simulink library "forward_dynamics_v1"  (R2020b)
settings: Solver=VariableStepAuto  StartTime=0.0  StopTime=10.0  RelTol=1e-3
undefined symbols (not defined in the file): Config, DiscIntNeverNeededParam
libraries: WBToolboxLibrary x21
settings Model: Creator=gnava  LastModifiedBy=gnava

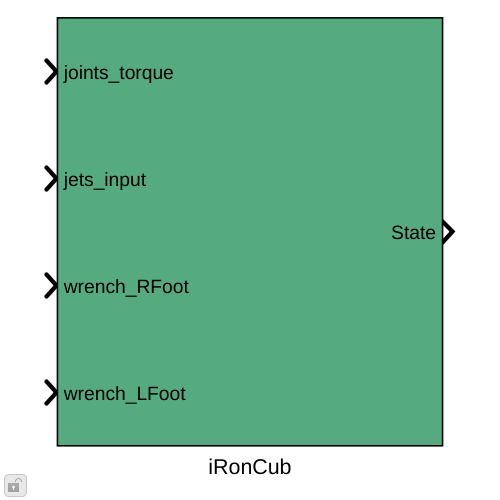
[thumbnail: Simulink's stored preview of the top-level diagram]
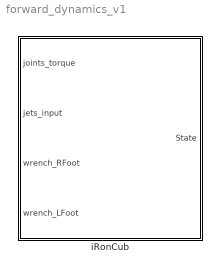
== system forward_dynamics_v1 ==
  iRonCub : Subsystem  mask{Config=Config}
      mask prompts: Config "Configuration structure"
      mask DialogControl DescTextVar Prompt: Block that simulates iRonCub

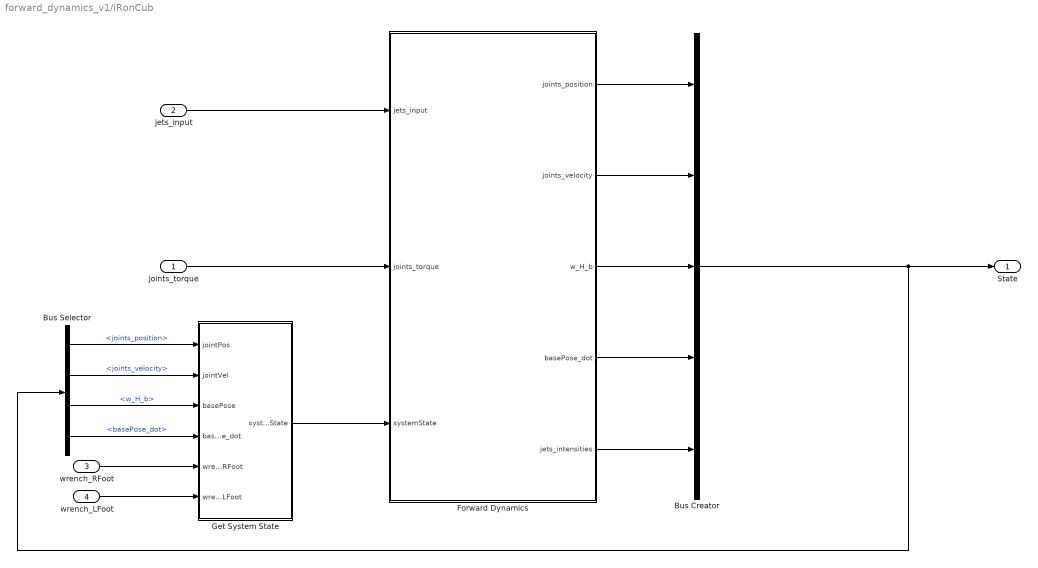
== system forward_dynamics_v1/iRonCub ==
  joints_torque : Inport
  jets_input : Inport  Port=2
  wrench_RFoot : Inport  Port=3
  wrench_LFoot : Inport  Port=4
  Bus Creator : BusCreator  Inputs=5
  Bus Selector : BusSelector  OutputSignals=joints_position,joints_velocity,w_H_b,basePose_dot
  Forward Dynamics : Subsystem
  Get System State : Subsystem
  State : Outport  VectorParamsAs1DForOutWhenUnconnected=off
  wires:
  jets_input/1 -> Forward Dynamics/1(jets_input)
  Get System State/1(systemState) -> Forward Dynamics/3(systemState)
  joints_torque/1 -> Forward Dynamics/2(joints_torque)
  Forward Dynamics/1(joints_position) -> Bus Creator/1
  Forward Dynamics/3(w_H_b) -> Bus Creator/3
  Forward Dynamics/4(basePose_dot) -> Bus Creator/4
  Bus Creator/1 -> State/1, Bus Selector/1
  Bus Selector/1 -> Get System State/1(jointPos)  "<joints_position>"
  Bus Selector/2 -> Get System State/2(jointVel)  "<joints_velocity>"
  Bus Selector/3 -> Get System State/3(basePose)  "<w_H_b>"
  Bus Selector/4 -> Get System State/4(basePose_dot)  "<basePose_dot>"
  wrench_RFoot/1 -> Get System State/5(wrench_RFoot)
  wrench_LFoot/1 -> Get System State/6(wrench_LFoot)
  Forward Dynamics/5(jets_intensities) -> Bus Creator/5
  Forward Dynamics/2(joints_velocity) -> Bus Creator/2

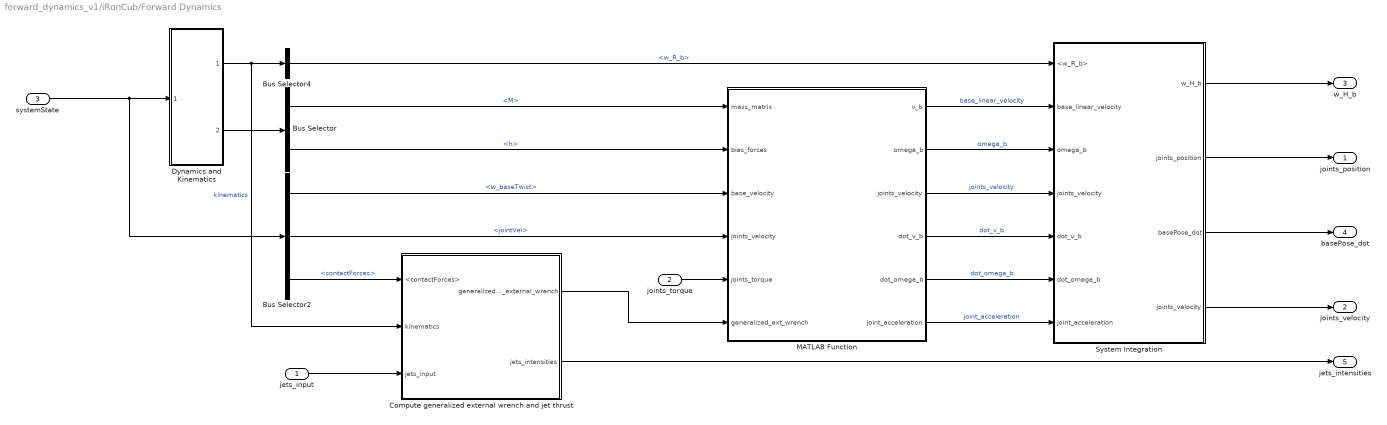
== system forward_dynamics_v1/iRonCub/Forward Dynamics ==
  jets_input : Inport
  joints_torque : Inport  Port=2
  systemState : Inport  Port=3
  Bus Selector : BusSelector  OutputSignals=M,h
  Bus Selector2 : BusSelector  OutputSignals=w_baseTwist,jointVel,contactForces
  Bus Selector4 : BusSelector  OutputSignals=w_R_b
  Compute generalized external wrench and jet thrust : Subsystem
  Dynamics and Kinematics : Subsystem
  MATLAB Function : MATLAB Function  TreatAsAtomicUnit=on
  System Integration : Subsystem
  joints_position : Outport  VectorParamsAs1DForOutWhenUnconnected=off
  joints_velocity : Outport  Port=2  VectorParamsAs1DForOutWhenUnconnected=off
  w_H_b : Outport  Port=3  VectorParamsAs1DForOutWhenUnconnected=off
  basePose_dot : Outport  Port=4  VectorParamsAs1DForOutWhenUnconnected=off
  jets_intensities : Outport  Port=5  VectorParamsAs1DForOutWhenUnconnected=off
  wires:
  Dynamics and Kinematics/1(kinematics) -> Compute generalized external wrench and jet thrust/2(kinematics), Bus Selector4/1  "kinematics"
  Bus Selector/2 -> MATLAB Function/2(bias_forces)  "<h>"
  Bus Selector/1 -> MATLAB Function/1(mass_matrix)  "<M>"
  Bus Selector2/1 -> MATLAB Function/3(base_velocity)  "<w_baseTwist>"
  Dynamics and Kinematics/2(dynamics) -> Bus Selector/1
  Bus Selector2/2 -> MATLAB Function/4("joints_velocity ")  "<jointVel>"
  systemState/1 -> Bus Selector2/1, Dynamics and Kinematics/1(systemState)
  MATLAB Function/1(v_b) -> System Integration/2(base_linear_velocity)  "base_linear_velocity"
  MATLAB Function/2(omega_b) -> System Integration/3(omega_b)  "omega_b"
  MATLAB Function/3(joints_velocity) -> System Integration/4(joints_velocity)  "joints_velocity"
  MATLAB Function/4(dot_v_b) -> System Integration/5(dot_v_b)  "dot_v_b"
  MATLAB Function/5(dot_omega_b) -> System Integration/6(dot_omega_b)  "dot_omega_b"
  MATLAB Function/6(joint_acceleration) -> System Integration/7(joint_acceleration)  "joint_acceleration"
  System Integration/1(w_H_b) -> w_H_b/1
  System Integration/2(joints_position) -> joints_position/1
  System Integration/3(basePose_dot) -> basePose_dot/1
  System Integration/4("joints_velocity ") -> joints_velocity/1
  Bus Selector4/1 -> System Integration/1(<w_R_b>)  "<w_R_b>"
  joints_torque/1 -> MATLAB Function/5(joints_torque)
  Bus Selector2/3 -> Compute generalized external wrench and jet thrust/1(<contactForces>)  "<contactForces>"
  jets_input/1 -> Compute generalized external wrench and jet thrust/3(jets_input)
  Compute generalized external wrench and jet thrust/1(generalized_external_wrench) -> MATLAB Function/6(generalized_ext_wrench)
  Compute generalized external wrench and jet thrust/2(jets_intensities) -> jets_intensities/1

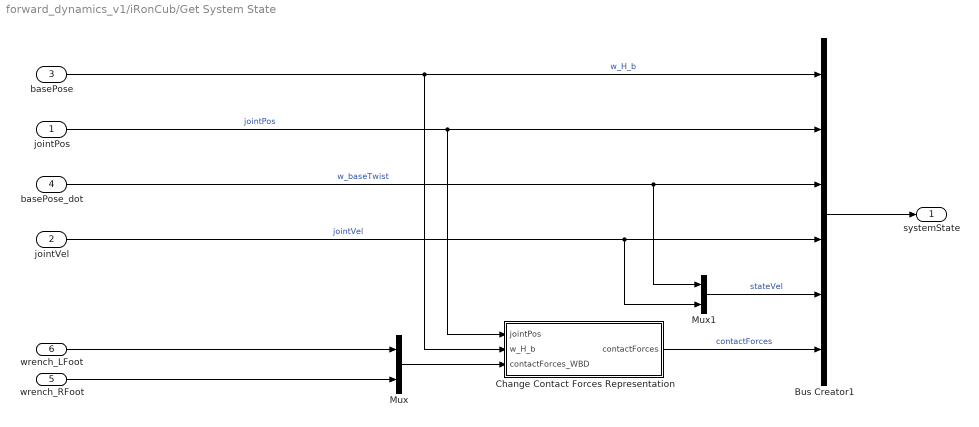
== system forward_dynamics_v1/iRonCub/Get System State ==
  jointPos : Inport
  jointVel : Inport  Port=2
  basePose : Inport  Port=3
  basePose_dot : Inport  Port=4
  wrench_RFoot : Inport  Port=5
  wrench_LFoot : Inport  Port=6
  Bus Creator1 : BusCreator  Inputs=6
  Change Contact Forces Representation : Subsystem
  Mux : Mux  Inputs=2
  Mux1 : Mux  Inputs=2
  systemState : Outport  VectorParamsAs1DForOutWhenUnconnected=off
  wires:
  wrench_LFoot/1 -> Mux/1
  wrench_RFoot/1 -> Mux/2
  Mux/1 -> Change Contact Forces Representation/3(contactForces_WBD)
  Change Contact Forces Representation/1(contactForces) -> Bus Creator1/6  "contactForces"
  jointVel/1 -> Bus Creator1/4, Mux1/2  "jointVel"
  Bus Creator1/1 -> systemState/1
  Mux1/1 -> Bus Creator1/5  "stateVel"
  basePose_dot/1 -> Bus Creator1/3, Mux1/1  "w_baseTwist"
  jointPos/1 -> Bus Creator1/2, Change Contact Forces Representation/1(jointPos)  "jointPos"
  basePose/1 -> Change Contact Forces Representation/2(w_H_b), Bus Creator1/1  "w_H_b"

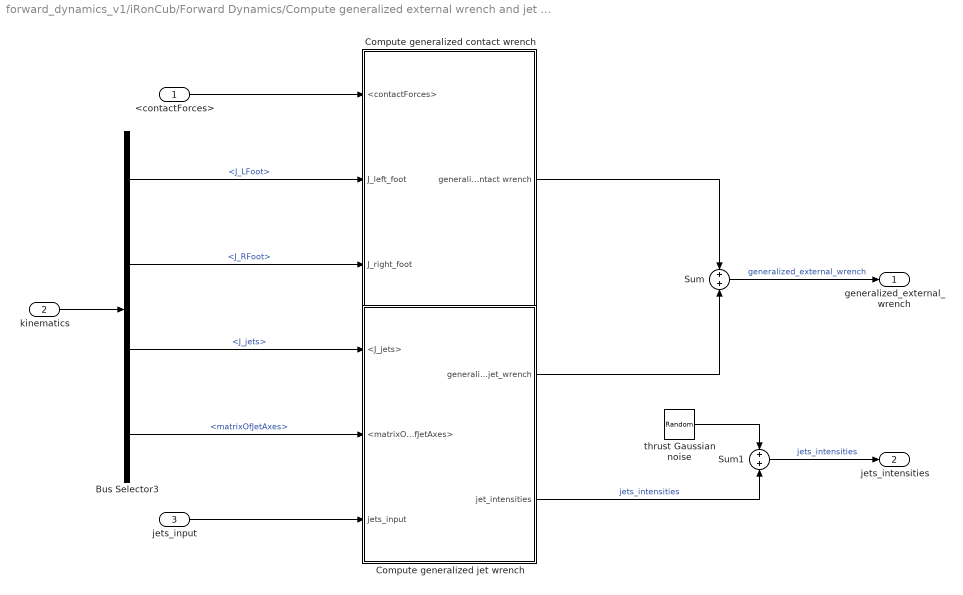
== system forward_dynamics_v1/iRonCub/Forward Dynamics/Compute generalized external wrench and jet thrust ==
  <contactForces> : Inport
  kinematics : Inport  Port=2
  jets_input : Inport  Port=3
  Bus Selector3 : BusSelector  OutputSignals=J_LFoot,J_RFoot,J_jets,matrixOfJetAxes
  "Compute generalized contact wrench " : Subsystem
  Compute generalized jet wrench : Subsystem
  Sum : Sum
  Sum1 : Sum
  "thrust Gaussian noise " : RandomNumber  Variance=Config.thrust_noise
  generalized_external_wrench : Outport  VectorParamsAs1DForOutWhenUnconnected=off
  jets_intensities : Outport  Port=2  VectorParamsAs1DForOutWhenUnconnected=off
  wires:
  Sum1/1 -> jets_intensities/1  "jets_intensities"
  "Compute generalized contact wrench "/1("generalized contact wrench ") -> Sum/1
  Bus Selector3/4 -> Compute generalized jet wrench/2(<matrixOfJetAxes>)  "<matrixOfJetAxes>"
  jets_input/1 -> Compute generalized jet wrench/3(jets_input)
  Bus Selector3/3 -> Compute generalized jet wrench/1(<J_jets>)  "<J_jets>"
  kinematics/1 -> Bus Selector3/1
  Compute generalized jet wrench/1(generalized_jet_wrench) -> Sum/2
  <contactForces>/1 -> "Compute generalized contact wrench "/1(<contactForces>)
  Sum/1 -> generalized_external_wrench/1  "generalized_external_wrench"
  Bus Selector3/1 -> "Compute generalized contact wrench "/2(J_left_foot)  "<J_LFoot>"
  Bus Selector3/2 -> "Compute generalized contact wrench "/3(J_right_foot)  "<J_RFoot>"
  "thrust Gaussian noise "/1 -> Sum1/1
  Compute generalized jet wrench/2(jet_intensities) -> Sum1/2  "jets_intensities"

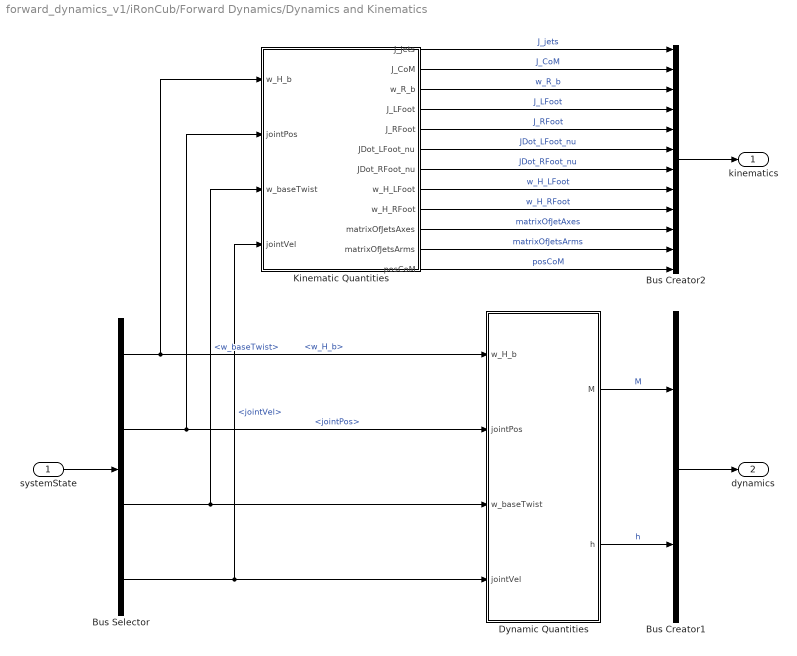
== system forward_dynamics_v1/iRonCub/Forward Dynamics/Dynamics and Kinematics ==
  systemState : Inport
  Bus Creator1 : BusCreator  Inputs=2
  Bus Creator2 : BusCreator  Inputs=12
  Bus Selector : BusSelector  OutputSignals=w_H_b,jointPos,w_baseTwist,jointVel
  Dynamic Quantities : Subsystem
  Kinematic Quantities : Subsystem
  kinematics : Outport  VectorParamsAs1DForOutWhenUnconnected=off
  dynamics : Outport  Port=2  VectorParamsAs1DForOutWhenUnconnected=off
  wires:
  systemState/1 -> Bus Selector/1
  Bus Selector/1 -> Dynamic Quantities/1(w_H_b), Kinematic Quantities/1(w_H_b)  "<w_H_b>"
  Bus Selector/2 -> Kinematic Quantities/2(jointPos), Dynamic Quantities/2(jointPos)  "<jointPos>"
  Bus Selector/3 -> Kinematic Quantities/3(w_baseTwist), Dynamic Quantities/3(w_baseTwist)  "<w_baseTwist>"
  Bus Selector/4 -> Kinematic Quantities/4(jointVel), Dynamic Quantities/4(jointVel)  "<jointVel>"
  Dynamic Quantities/2("h ") -> Bus Creator1/2  "h"
  Dynamic Quantities/1(M) -> Bus Creator1/1  "M"
  Bus Creator1/1 -> dynamics/1
  Bus Creator2/1 -> kinematics/1
  Kinematic Quantities/1(J_jets) -> Bus Creator2/1  "J_jets"
  Kinematic Quantities/2(J_CoM) -> Bus Creator2/2  "J_CoM"
  Kinematic Quantities/3(w_R_b) -> Bus Creator2/3  "w_R_b"
  Kinematic Quantities/4(J_LFoot) -> Bus Creator2/4  "J_LFoot"
  Kinematic Quantities/5(J_RFoot) -> Bus Creator2/5  "J_RFoot"
  Kinematic Quantities/6(JDot_LFoot_nu) -> Bus Creator2/6  "JDot_LFoot_nu"
  Kinematic Quantities/7(JDot_RFoot_nu) -> Bus Creator2/7  "JDot_RFoot_nu"
  Kinematic Quantities/8(w_H_LFoot) -> Bus Creator2/8  "w_H_LFoot"
  Kinematic Quantities/9(w_H_RFoot) -> Bus Creator2/9  "w_H_RFoot"
  Kinematic Quantities/10(matrixOfJetsAxes) -> Bus Creator2/10  "matrixOfJetAxes"
  Kinematic Quantities/11(matrixOfJetsArms) -> Bus Creator2/11  "matrixOfJetsArms"
  Kinematic Quantities/12(posCoM) -> Bus Creator2/12  "posCoM"

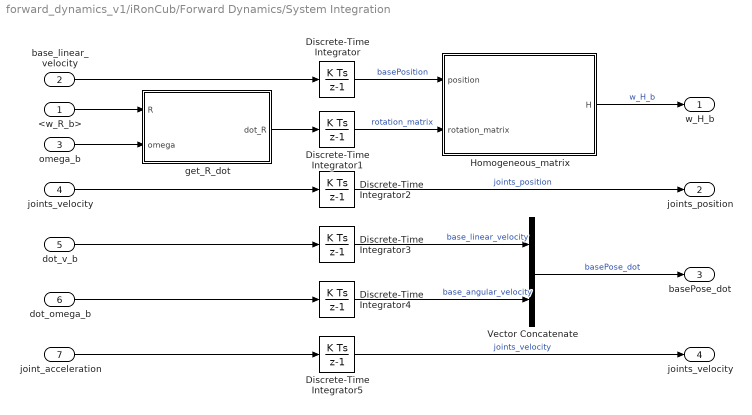
== system forward_dynamics_v1/iRonCub/Forward Dynamics/System Integration ==
  <w_R_b> : Inport
  base_linear_velocity : Inport  Port=2
  omega_b : Inport  Port=3
  joints_velocity : Inport  Port=4
  dot_v_b : Inport  Port=5
  dot_omega_b : Inport  Port=6
  joint_acceleration : Inport  Port=7
  Discrete-Time Integrator : DiscreteIntegrator  InitialCondition=Config.initialConditions.base_position  SampleTime=-1  ICPrevOutput=DiscIntNeverNeededParam  ICPrevScaledInput=DiscIntNeverNeededParam
  Discrete-Time Integrator1 : DiscreteIntegrator  InitialCondition=Config.initialConditions.orientation  SampleTime=-1  ICPrevOutput=DiscIntNeverNeededParam  ICPrevScaledInput=DiscIntNeverNeededParam
  Discrete-Time Integrator2 : DiscreteIntegrator  InitialCondition=Config.initialConditions.joints  SampleTime=-1  ICPrevOutput=DiscIntNeverNeededParam  ICPrevScaledInput=DiscIntNeverNeededParam
  Discrete-Time Integrator3 : DiscreteIntegrator  InitialCondition=Config.initialConditions.base_linear_velocity  SampleTime=-1  ICPrevOutput=DiscIntNeverNeededParam  ICPrevScaledInput=DiscIntNeverNeededParam
  Discrete-Time Integrator4 : DiscreteIntegrator  InitialCondition=Config.initialConditions.base_angular_velocity  SampleTime=-1  ICPrevOutput=DiscIntNeverNeededParam  ICPrevScaledInput=DiscIntNeverNeededParam
  Discrete-Time Integrator5 : DiscreteIntegrator  InitialCondition=Config.initialConditions.joints_velocity  SampleTime=-1  ICPrevOutput=DiscIntNeverNeededParam  ICPrevScaledInput=DiscIntNeverNeededParam
  "Homogeneous_matrix " : MATLAB Function  TreatAsAtomicUnit=on
  Vector Concatenate : Concatenate
  "get_R_dot " : MATLAB Function  TreatAsAtomicUnit=on
  w_H_b : Outport  VectorParamsAs1DForOutWhenUnconnected=off
  joints_position : Outport  Port=2  VectorParamsAs1DForOutWhenUnconnected=off
  basePose_dot : Outport  Port=3  VectorParamsAs1DForOutWhenUnconnected=off
  "joints_velocity " : Outport  Port=4  VectorParamsAs1DForOutWhenUnconnected=off
  wires:
  Discrete-Time Integrator3/1 -> Vector Concatenate/1  "base_linear_velocity"
  omega_b/1 -> "get_R_dot "/2(omega)
  Discrete-Time Integrator5/1 -> "joints_velocity "/1  "joints_velocity"
  dot_v_b/1 -> Discrete-Time Integrator3/1
  Discrete-Time Integrator2/1 -> joints_position/1  "joints_position"
  <w_R_b>/1 -> "get_R_dot "/1(R)
  Discrete-Time Integrator4/1 -> Vector Concatenate/2  "base_angular_velocity"
  "Homogeneous_matrix "/1(H) -> w_H_b/1  "w_H_b"
  Vector Concatenate/1 -> basePose_dot/1  "basePose_dot"
  joints_velocity/1 -> Discrete-Time Integrator2/1
  Discrete-Time Integrator/1 -> "Homogeneous_matrix "/1(position)  "basePosition"
  base_linear_velocity/1 -> Discrete-Time Integrator/1
  "get_R_dot "/1(dot_R) -> Discrete-Time Integrator1/1
  dot_omega_b/1 -> Discrete-Time Integrator4/1
  joint_acceleration/1 -> Discrete-Time Integrator5/1
  Discrete-Time Integrator1/1 -> "Homogeneous_matrix "/2(rotation_matrix)  "rotation_matrix"

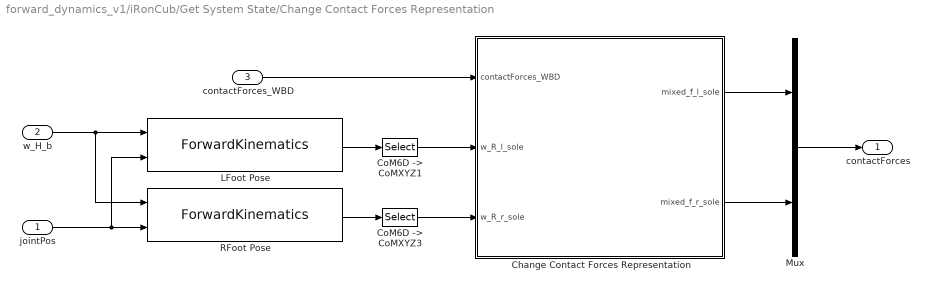
== system forward_dynamics_v1/iRonCub/Get System State/Change Contact Forces Representation ==
  jointPos : Inport
  w_H_b : Inport  Port=2
  contactForces_WBD : Inport  Port=3
  Change Contact Forces Representation : MATLAB Function  TreatAsAtomicUnit=on
  "CoM6D -> CoMXYZ1" : Selector  NumberOfDimensions=2  InputPortWidth=7  IndexOptions=Index vector (dialog),Index vector (dialog)  Indices=[1 2 3],[1 2 3]  OutputSizes=1,1
  "CoM6D -> CoMXYZ3" : Selector  NumberOfDimensions=2  InputPortWidth=7  IndexOptions=Index vector (dialog),Index vector (dialog)  Indices=[1 2 3],[1 2 3]  OutputSizes=1,1
  LFoot Pose : WBToolboxLibrary/Model/Kinematics/ForwardKinematics  frameName=Frames.LFOOT_FRAME
      settings: SourceProductName=WholeBodyToolbox
  Mux : Mux  Inputs=2
  RFoot Pose : WBToolboxLibrary/Model/Kinematics/ForwardKinematics  frameName=Frames.RFOOT_FRAME
      settings: SourceProductName=WholeBodyToolbox
  contactForces : Outport  VectorParamsAs1DForOutWhenUnconnected=off
  wires:
  contactForces_WBD/1 -> Change Contact Forces Representation/1(contactForces_WBD)
  RFoot Pose/1 -> "CoM6D -> CoMXYZ3"/1
  "CoM6D -> CoMXYZ3"/1 -> Change Contact Forces Representation/3(w_R_r_sole)
  LFoot Pose/1 -> "CoM6D -> CoMXYZ1"/1
  "CoM6D -> CoMXYZ1"/1 -> Change Contact Forces Representation/2(w_R_l_sole)
  w_H_b/1 -> LFoot Pose/1, RFoot Pose/1
  jointPos/1 -> LFoot Pose/2, RFoot Pose/2
  Change Contact Forces Representation/1(mixed_f_l_sole) -> Mux/1
  Change Contact Forces Representation/2(mixed_f_r_sole) -> Mux/2
  Mux/1 -> contactForces/1

== system forward_dynamics_v1/iRonCub/Forward Dynamics/Compute generalized external wrench and jet thrust/Compute generalized contact wrench  ==
  <contactForces> : Inport
  J_left_foot : Inport  Port=2
  J_right_foot : Inport  Port=3
  Matrix Concatenate : Concatenate  Mode=Multidimensional array
  MatrixMultiply : Product  Multiplication=Matrix(*)
  Transpose : Math  Operator=transpose  SignedPower=on  SaturateOnIntegerOverflow=on
  "generalized contact wrench " : Outport  VectorParamsAs1DForOutWhenUnconnected=off
  wires:
  J_left_foot/1 -> Matrix Concatenate/1
  J_right_foot/1 -> Matrix Concatenate/2
  Matrix Concatenate/1 -> Transpose/1
  <contactForces>/1 -> MatrixMultiply/2
  Transpose/1 -> MatrixMultiply/1
  MatrixMultiply/1 -> "generalized contact wrench "/1

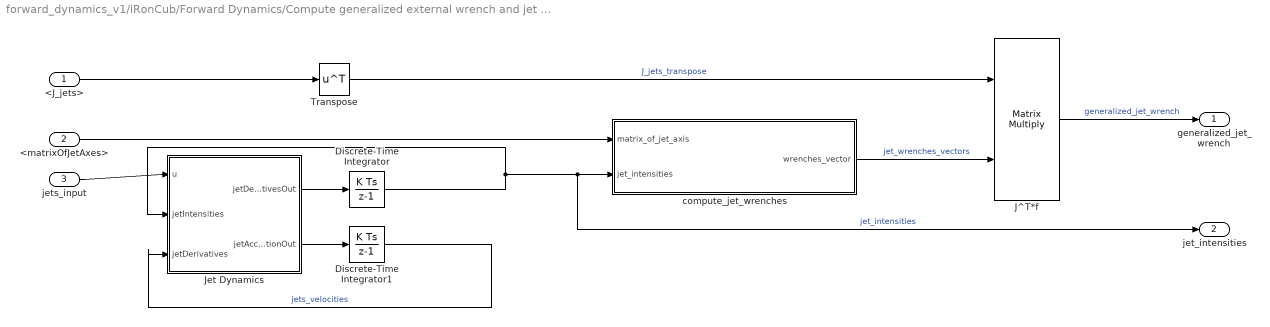
== system forward_dynamics_v1/iRonCub/Forward Dynamics/Compute generalized external wrench and jet thrust/Compute generalized jet wrench ==
  <J_jets> : Inport
  <matrixOfJetAxes> : Inport  Port=2
  jets_input : Inport  Port=3
  Discrete-Time Integrator : DiscreteIntegrator  InitialCondition=Config.initialConditions.jets_thrust  SampleTime=-1  ICPrevOutput=DiscIntNeverNeededParam  ICPrevScaledInput=DiscIntNeverNeededParam
  Discrete-Time Integrator1 : DiscreteIntegrator  SampleTime=-1  ICPrevOutput=DiscIntNeverNeededParam  ICPrevScaledInput=DiscIntNeverNeededParam
  J^T*f : Product  Multiplication=Matrix(*)
  Jet Dynamics : MATLAB Function  TreatAsAtomicUnit=on
  Transpose : Math  Operator=transpose  SignedPower=on  SaturateOnIntegerOverflow=on
  "compute_jet_wrenches " : MATLAB Function  TreatAsAtomicUnit=on
  generalized_jet_wrench : Outport  VectorParamsAs1DForOutWhenUnconnected=off
  jet_intensities : Outport  Port=2  VectorParamsAs1DForOutWhenUnconnected=off
  wires:
  "compute_jet_wrenches "/1(wrenches_vector) -> J^T*f/2  "jet_wrenches_vectors"
  <matrixOfJetAxes>/1 -> "compute_jet_wrenches "/1(matrix_of_jet_axis)
  Transpose/1 -> J^T*f/1  "J_jets_transpose"
  <J_jets>/1 -> Transpose/1
  jets_input/1 -> Jet Dynamics/1(u)
  Discrete-Time Integrator/1 -> jet_intensities/1, "compute_jet_wrenches "/2(jet_intensities), Jet Dynamics/2(jetIntensities)  "jet_intensities"
  J^T*f/1 -> generalized_jet_wrench/1  "generalized_jet_wrench"
  Jet Dynamics/2(jetAccelerationOut) -> Discrete-Time Integrator1/1
  Discrete-Time Integrator1/1 -> Jet Dynamics/3(jetDerivatives)  "jets_velocities"
  Jet Dynamics/1(jetDerivativesOut) -> Discrete-Time Integrator/1

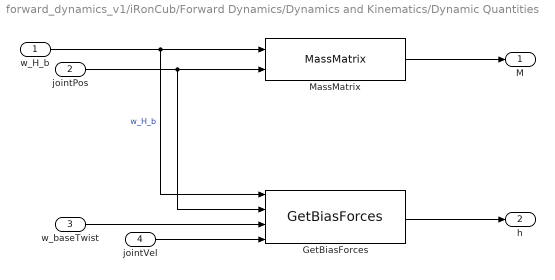
== system forward_dynamics_v1/iRonCub/Forward Dynamics/Dynamics and Kinematics/Dynamic Quantities ==
  w_H_b : Inport
  jointPos : Inport  Port=2
  w_baseTwist : Inport  Port=3
  jointVel : Inport  Port=4
  GetBiasForces : WBToolboxLibrary/Model/Dynamics/GetBiasForces
      settings: SourceProductName=WholeBodyToolbox
  MassMatrix : WBToolboxLibrary/Model/Dynamics/MassMatrix
      settings: SourceProductName=WholeBodyToolbox
  M : Outport  VectorParamsAs1DForOutWhenUnconnected=off
  "h " : Outport  Port=2  VectorParamsAs1DForOutWhenUnconnected=off
  wires:
  w_H_b/1 -> GetBiasForces/1, MassMatrix/1  "w_H_b"
  w_baseTwist/1 -> GetBiasForces/3
  jointVel/1 -> GetBiasForces/4
  MassMatrix/1 -> M/1
  GetBiasForces/1 -> "h "/1
  jointPos/1 -> GetBiasForces/2, MassMatrix/2

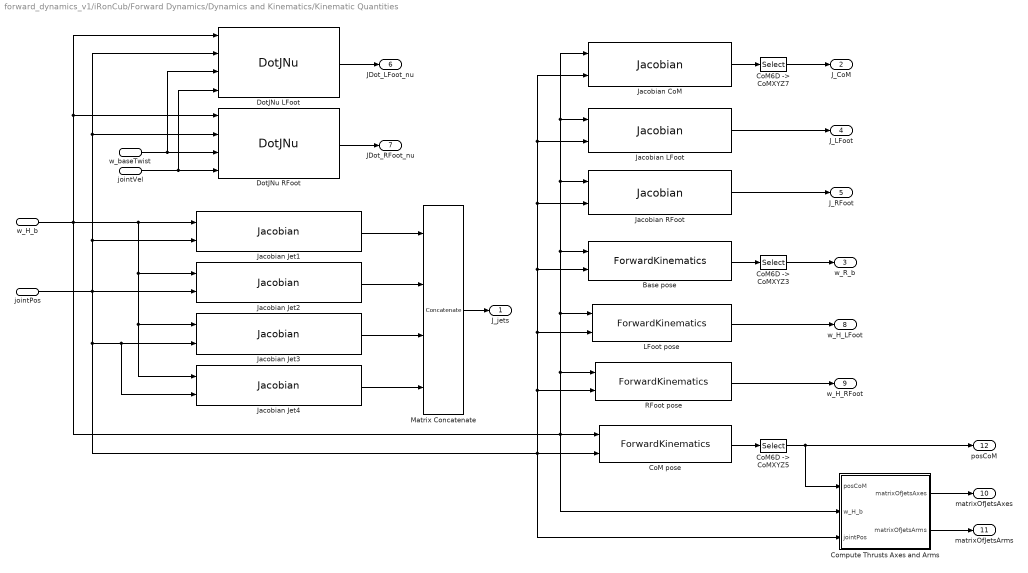
== system forward_dynamics_v1/iRonCub/Forward Dynamics/Dynamics and Kinematics/Kinematic Quantities ==
  w_H_b : Inport
  jointPos : Inport  Port=2
  w_baseTwist : Inport  Port=3
  jointVel : Inport  Port=4
  Base pose : WBToolboxLibrary/Model/Kinematics/ForwardKinematics  frameName=Frames.BASE_LINK
      settings: SourceProductName=WholeBodyToolbox
  CoM pose : WBToolboxLibrary/Model/Kinematics/ForwardKinematics  frameName=Frames.COM_FRAME
      settings: SourceProductName=WholeBodyToolbox
  "CoM6D -> CoMXYZ3" : Selector  NumberOfDimensions=2  InputPortWidth=7  IndexOptions=Index vector (dialog),Index vector (dialog)  Indices=[1 2 3],[1 2 3]  OutputSizes=1,1
  "CoM6D -> CoMXYZ5" : Selector  NumberOfDimensions=2  InputPortWidth=7  IndexOptions=Index vector (dialog),Index vector (dialog)  Indices=[1 2 3],[4]  OutputSizes=1,1
  "CoM6D -> CoMXYZ7" : Selector  NumberOfDimensions=2  InputPortWidth=7  IndexOptions=Index vector (dialog),Index vector (dialog)  Indices=[1 2 3],[1:6+Config.N_DOF]  OutputSizes=1,1
  Compute Thrusts Axes and Arms : Subsystem
  DotJNu LFoot : WBToolboxLibrary/Model/Jacobians/DotJNu  frameName=Frames.LFOOT_FRAME
      settings: SourceProductName=WholeBodyToolbox
  DotJNu RFoot : WBToolboxLibrary/Model/Jacobians/DotJNu  frameName=Frames.RFOOT_FRAME
      settings: SourceProductName=WholeBodyToolbox
  Jacobian CoM : WBToolboxLibrary/Model/Jacobians/Jacobian  frameName=Frames.COM_FRAME
      settings: SourceProductName=WholeBodyToolbox
  Jacobian Jet1 : WBToolboxLibrary/Model/Jacobians/Jacobian  frameName=Frames.JET1_FRAME
      settings: SourceProductName=WholeBodyToolbox
  Jacobian Jet2 : WBToolboxLibrary/Model/Jacobians/Jacobian  frameName=Frames.JET2_FRAME
      settings: SourceProductName=WholeBodyToolbox
  Jacobian Jet3 : WBToolboxLibrary/Model/Jacobians/Jacobian  frameName=Frames.JET3_FRAME
      settings: SourceProductName=WholeBodyToolbox
  Jacobian Jet4 : WBToolboxLibrary/Model/Jacobians/Jacobian  frameName=Frames.JET4_FRAME
      settings: SourceProductName=WholeBodyToolbox
  Jacobian LFoot : WBToolboxLibrary/Model/Jacobians/Jacobian  frameName=Frames.LFOOT_FRAME
      settings: SourceProductName=WholeBodyToolbox
  Jacobian RFoot : WBToolboxLibrary/Model/Jacobians/Jacobian  frameName=Frames.RFOOT_FRAME
      settings: SourceProductName=WholeBodyToolbox
  LFoot pose : WBToolboxLibrary/Model/Kinematics/ForwardKinematics  frameName=Frames.LFOOT_FRAME
      settings: SourceProductName=WholeBodyToolbox
  Matrix Concatenate : Concatenate  NumInputs=4  Mode=Multidimensional array
  RFoot pose : WBToolboxLibrary/Model/Kinematics/ForwardKinematics  frameName=Frames.RFOOT_FRAME
      settings: SourceProductName=WholeBodyToolbox
  J_jets : Outport  VectorParamsAs1DForOutWhenUnconnected=off
  J_CoM : Outport  Port=2  VectorParamsAs1DForOutWhenUnconnected=off
  w_R_b : Outport  Port=3  VectorParamsAs1DForOutWhenUnconnected=off
  J_LFoot : Outport  Port=4  VectorParamsAs1DForOutWhenUnconnected=off
  J_RFoot : Outport  Port=5  VectorParamsAs1DForOutWhenUnconnected=off
  JDot_LFoot_nu : Outport  Port=6  VectorParamsAs1DForOutWhenUnconnected=off
  JDot_RFoot_nu : Outport  Port=7  VectorParamsAs1DForOutWhenUnconnected=off
  w_H_LFoot : Outport  Port=8  VectorParamsAs1DForOutWhenUnconnected=off
  w_H_RFoot : Outport  Port=9  VectorParamsAs1DForOutWhenUnconnected=off
  matrixOfJetsAxes : Outport  Port=10  VectorParamsAs1DForOutWhenUnconnected=off
  matrixOfJetsArms : Outport  Port=11  VectorParamsAs1DForOutWhenUnconnected=off
  posCoM : Outport  Port=12  VectorParamsAs1DForOutWhenUnconnected=off
  wires:
  Matrix Concatenate/1 -> J_jets/1
  CoM pose/1 -> "CoM6D -> CoMXYZ5"/1
  "CoM6D -> CoMXYZ5"/1 -> posCoM/1, Compute Thrusts Axes and Arms/1(posCoM)
  w_H_b/1 -> LFoot pose/1, Base pose/1, Jacobian LFoot/1, Jacobian CoM/1, Jacobian RFoot/1, RFoot pose/1, CoM pose/1, Compute Thrusts Axes and Arms/2(w_H_b), DotJNu LFoot/1, DotJNu RFoot/1, Jacobian Jet4/1, Jacobian Jet3/1, Jacobian Jet2/1, Jacobian Jet1/1
  "CoM6D -> CoMXYZ3"/1 -> w_R_b/1
  jointPos/1 -> Jacobian Jet4/2, Jacobian Jet3/2, Compute Thrusts Axes and Arms/3(jointPos), LFoot pose/2, Jacobian RFoot/2, Jacobian LFoot/2, Jacobian CoM/2, Base pose/2, RFoot pose/2, CoM pose/2, Jacobian Jet2/2, DotJNu LFoot/2, DotJNu RFoot/2, Jacobian Jet1/2
  Jacobian CoM/1 -> "CoM6D -> CoMXYZ7"/1
  Jacobian RFoot/1 -> J_RFoot/1
  Jacobian LFoot/1 -> J_LFoot/1
  DotJNu RFoot/1 -> JDot_RFoot_nu/1
  DotJNu LFoot/1 -> JDot_LFoot_nu/1
  jointVel/1 -> DotJNu RFoot/4, DotJNu LFoot/4
  w_baseTwist/1 -> DotJNu LFoot/3, DotJNu RFoot/3
  RFoot pose/1 -> w_H_RFoot/1
  LFoot pose/1 -> w_H_LFoot/1
  Base pose/1 -> "CoM6D -> CoMXYZ3"/1
  Compute Thrusts Axes and Arms/2(matrixOfJetsArms) -> matrixOfJetsArms/1
  Compute Thrusts Axes and Arms/1(matrixOfJetsAxes) -> matrixOfJetsAxes/1
  Jacobian Jet1/1 -> Matrix Concatenate/1
  Jacobian Jet2/1 -> Matrix Concatenate/2
  Jacobian Jet3/1 -> Matrix Concatenate/3
  Jacobian Jet4/1 -> Matrix Concatenate/4
  "CoM6D -> CoMXYZ7"/1 -> J_CoM/1

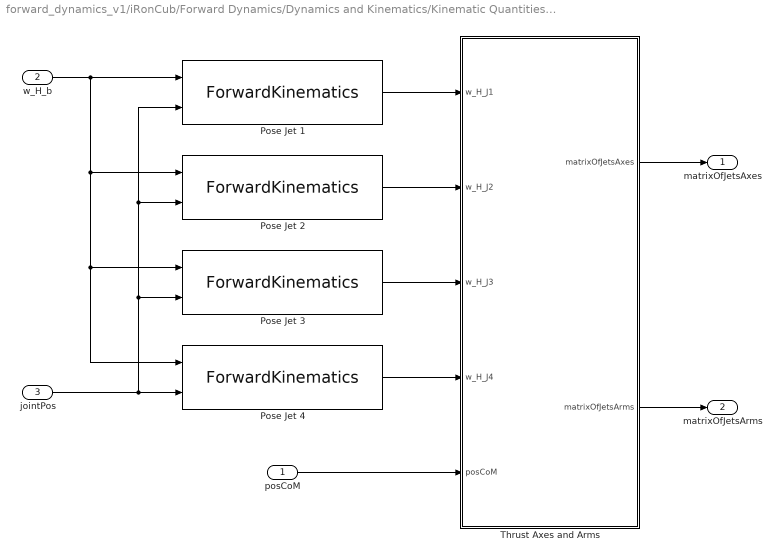
== system forward_dynamics_v1/iRonCub/Forward Dynamics/Dynamics and Kinematics/Kinematic Quantities/Compute Thrusts Axes and Arms ==
  posCoM : Inport
  w_H_b : Inport  Port=2
  jointPos : Inport  Port=3
  Pose Jet 1 : WBToolboxLibrary/Model/Kinematics/ForwardKinematics  frameName=Frames.JET1_FRAME
      settings: SourceProductName=WholeBodyToolbox
  Pose Jet 2 : WBToolboxLibrary/Model/Kinematics/ForwardKinematics  frameName=Frames.JET2_FRAME
      settings: SourceProductName=WholeBodyToolbox
  Pose Jet 3 : WBToolboxLibrary/Model/Kinematics/ForwardKinematics  frameName=Frames.JET3_FRAME
      settings: SourceProductName=WholeBodyToolbox
  Pose Jet 4 : WBToolboxLibrary/Model/Kinematics/ForwardKinematics  frameName=Frames.JET4_FRAME
      settings: SourceProductName=WholeBodyToolbox
  Thrust Axes and Arms : MATLAB Function  TreatAsAtomicUnit=on
  matrixOfJetsAxes : Outport  VectorParamsAs1DForOutWhenUnconnected=off
  matrixOfJetsArms : Outport  Port=2  VectorParamsAs1DForOutWhenUnconnected=off
  wires:
  Pose Jet 2/1 -> Thrust Axes and Arms/2(w_H_J2)
  jointPos/1 -> Pose Jet 1/2, Pose Jet 2/2, Pose Jet 3/2, Pose Jet 4/2
  Pose Jet 1/1 -> Thrust Axes and Arms/1(w_H_J1)
  Pose Jet 3/1 -> Thrust Axes and Arms/3(w_H_J3)
  Pose Jet 4/1 -> Thrust Axes and Arms/4(w_H_J4)
  Thrust Axes and Arms/1(matrixOfJetsAxes) -> matrixOfJetsAxes/1
  Thrust Axes and Arms/2(matrixOfJetsArms) -> matrixOfJetsArms/1
  w_H_b/1 -> Pose Jet 4/1, Pose Jet 3/1, Pose Jet 2/1, Pose Jet 1/1
  posCoM/1 -> Thrust Axes and Arms/5(posCoM)

== matlab function forward_dynamics_v1/iRonCub/Forward Dynamics/MATLAB Function ==
  data: mass_matrix input size=[Config.N_DOF+6, Config.N_DOF+6]; bias_forces input size=[Config.N_DOF+6,1]; base_velocity input size=[6,1]; v_b output size=[3,1]; joints_velocity input size=[Config.N_DOF,1]; joints_torque input size=[Config.N_DOF,1]; generalized_ext_wrench input size=[Config.N_DOF+6,1]; Config parameter; omega_b output size=[3,1]; joints_velocity output; dot_v_b output size=[3,1]; dot_omega_b output size=[3,1]; joint_acceleration output size=[Config.N_DOF,1]
function [v_b, omega_b, joints_velocity, dot_v_b, dot_omega_b, joint_acceleration] ...
    = forwardDynamics(mass_matrix, bias_forces, base_velocity, joints_velocity, joints_torque, generalized_ext_wrench, Config)

[v_b, omega_b, joints_velocity, dot_v_b, dot_omega_b, joint_acceleration] ...
    = forwardDynamics(mass_matrix, bias_forces, base_velocity, joints_velocity, joints_torque, generalized_ext_wrench, Config);
end

== matlab function forward_dynamics_v1/iRonCub/Forward Dynamics/Compute generalized external wrench and jet thrust/Compute generalized jet wrench/Jet Dynamics ==
  data: u input; jetDerivativesOut output; jetIntensities input size=[4,1]; jetDerivatives input size=[4,1]; Config parameter; jetAccelerationOut output
function [jetDerivativesOut, jetAccelerationOut] = fcn(u, jetIntensities, jetDerivatives, Config)
jetDerivativesOut = zeros(4,1);
jetAccelerationOut = zeros(4,1);
for i=1:4
    state = [jetIntensities(i), jetDerivatives(i)];
    x = jetModel.get_xDot(state, Config.jet.coeff(i,:), u(i));
    jetDerivativesOut(i) = x(1);
    jetAccelerationOut(i) = x(2);
end
end

== matlab function forward_dynamics_v1/iRonCub/Forward Dynamics/Dynamics and Kinematics/Kinematic Quantities/Compute Thrusts Axes and Arms/Thrust Axes and Arms ==
  data: w_H_J1 input; matrixOfJetsAxes output; w_H_J2 input; w_H_J3 input; w_H_J4 input; posCoM input; matrixOfJetsArms output; Config parameter
function [matrixOfJetsAxes, matrixOfJetsArms] = computeJetsAxesAndArmsFCN(w_H_J1, w_H_J2, w_H_J3, w_H_J4, posCoM, Config)

    [matrixOfJetsAxes, matrixOfJetsArms] = computeJetsAxesAndArms(w_H_J1, w_H_J2, w_H_J3, w_H_J4, posCoM, Config);
end

== matlab function forward_dynamics_v1/iRonCub/Get System State/Change Contact Forces Representation/Change Contact Forces Representation ==
  data: contactForces_WBD input; mixed_f_l_sole output; w_R_l_sole input; w_R_r_sole input; mixed_f_r_sole output
function [mixed_f_l_sole, mixed_f_r_sole] = fromBodyFrameToMixed_contactForcesFCN(contactForces_WBD, w_R_l_sole, w_R_r_sole)

    [mixed_f_l_sole, mixed_f_r_sole] = fromBodyFrameToMixed_contactForces(contactForces_WBD, w_R_l_sole, w_R_r_sole);
end

== matlab function forward_dynamics_v1/iRonCub/Forward Dynamics/Compute generalized external wrench and jet thrust/Compute generalized jet wrench/compute_jet_wrenches  ==
  data: matrix_of_jet_axis input; wrenches_vector output; jet_intensities input
function wrenches_vector = compute_jet_wrenches(matrix_of_jet_axis, jet_intensities)
dim_wrench = 6;
num_jets = 4;

% the jets produce pure force (no momentum)
% the wrench is a 6dim vector [Fx, Fy, Fz, 0, 0, 0].transpose

wrenches_vector = zeros(dim_wrench*num_jets, 1);
for i=0:(num_jets-1)
    wrenches_vector(dim_wrench*i + 1: dim_wrench*i + dim_wrench/2) = matrix_of_jet_axis(:,i+1)*jet_intensities(i+1);
end

== matlab function forward_dynamics_v1/iRonCub/Forward Dynamics/System Integration/get_R_dot  ==
  data: R input; omega input; dot_R output
function dot_R = get_R_dot(R, omega)
% \dot{A_R_B} = S(omega_A)*A_R_B
% dot_R = wbc.skew(omega)*R;

gain = 0.001;
A = gain * ((R' * R)' - eye(3));

dot_R  = (wbc.skew(omega) + A) * R;

== matlab function forward_dynamics_v1/iRonCub/Forward Dynamics/System Integration/Homogeneous_matrix  ==
  data: position input; H output; rotation_matrix input
function H = homogeneous_matrix(position, rotation_matrix)
H = eye(4,4);
if abs(det(rotation_matrix) - 1) > 0.01
%     error('The rotation matrix is not a anymore a rotation matrix');
    disp('Making the matrix a rotation one using SVD');
    [U,~,V] = svd(rotation_matrix);
    rotation_matrix = U*V';
end
H(1:3,1:3) = rotation_matrix;
H(1:3,4) = position;
